simulink model "SMC"  (R2023b)
settings: Solver=VariableStepAuto  StartTime=0.0  StopTime=tf  RelTol=1e-7
values from neighbouring files (symbols this model uses):
  A = Ixx-Kpdot    (= 4100300)    [ShipFinStabilizers.m]
  b = B/A    (= -0.123183501573)    [ShipFinStabilizers.m]    (also in analisi_LUCIA.m = 1)
  B = Kp + Kup - 2*Kalpha*rf/U    (= -505089.3115)    [ShipFinStabilizers.m]
  c = C/A    (= -0.101455991025)    [ShipFinStabilizers.m]
  C = Knl    (= -416000)    [ShipFinStabilizers.m]
  controller_on = 1    [ShipFinStabilizers.m]    (also in off.m = 0; on.m; plotRoutine.m)
  d = D/A    (= -0.0647513596566)    [ShipFinStabilizers.m]    (also in analisi_LUCIA.m = -0.1)
  D = KphiUU*U^2    (= -265500)    [ShipFinStabilizers.m]
  f = F/A    (= -0.00439842816379)    [ShipFinStabilizers.m]
  F = -2*Kalpha    (= -18034.875)    [ShipFinStabilizers.m]
  Fw = 0.2    [ShipFinStabilizers.m]    (also in plotRoutine.m = Fw_vect(i))
  k = 8    [ShipFinStabilizers.m]    (also in analisi_LUCIA.m = 0.25)
  omega_w = 1.3    [ShipFinStabilizers.m]    (also in plotRoutine.m = omega_w_vect(j))
  p1 = 1    [ShipFinStabilizers.m]
  p2 = 2    [ShipFinStabilizers.m]
  rate = 90    [ShipFinStabilizers.m]
  regularizer = 0.1    [ShipFinStabilizers.m]
  sat = 45    [ShipFinStabilizers.m]
  x0 = [deg2rad(20);0]    [ShipFinStabilizers.m]
libraries: simulink x1
settings Model: Creator=valen  LastModifiedBy=valen

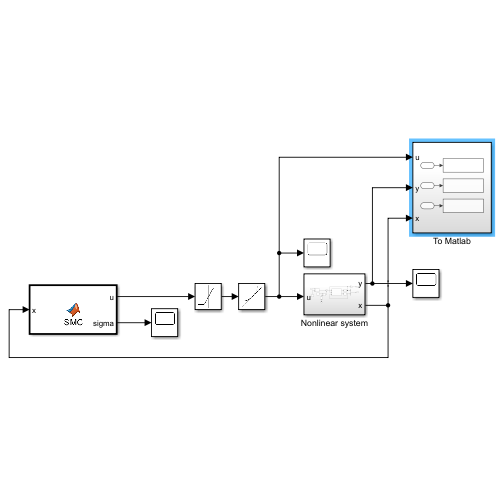
[thumbnail: Simulink's stored preview of the top-level diagram]
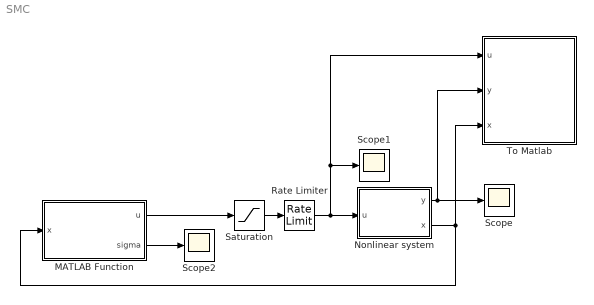
== system SMC ==
  MATLAB Function : MATLAB Function  TreatAsAtomicUnit=on
  Nonlinear system : Subsystem
  Rate Limiter : RateLimiter  RisingSlewLimit=rate  FallingSlewLimit=-rate  SampleTimeMode=inherited
  Saturation : Saturate  UpperLimit=sat  LowerLimit=-sat
  Scope : Scope
  Scope1 : Scope
  Scope2 : Scope
  To Matlab : Subsystem
  wires:
  Rate Limiter/1 -> Scope1/1, To Matlab/1(u), Nonlinear system/1(u)
  Saturation/1 -> Rate Limiter/1
  Nonlinear system/2(x) -> To Matlab/3(x), MATLAB Function/1(x)
  Nonlinear system/1(y) -> To Matlab/2(y), Scope/1
  MATLAB Function/1(u) -> Saturation/1
  MATLAB Function/2(sigma) -> Scope2/1

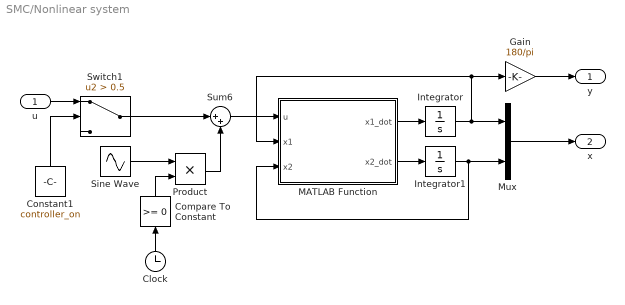
== system SMC/Nonlinear system ==
  u : Inport
  Clock : Clock
  Compare To Constant : simulink/Logic and Bit Operations/Compare To Constant  relop=>=  const=0  OutDataTypeStr=boolean
  Constant1 : Constant  Value=controller_on
  Gain : Gain  Gain=180/pi
  Integrator : Integrator  InitialCondition=x0(1)
  Integrator1 : Integrator  InitialCondition=x0(2)
  MATLAB Function : MATLAB Function  TreatAsAtomicUnit=on
  Mux : Mux  Inputs=2
  Product : Product
  Sine Wave : Sin  Amplitude=Fw/F*A  Frequency=omega_w  SampleTime=0
  Sum6 : Sum  Inputs=|++
  Switch1 : Switch  Criteria=u2 > Threshold  Threshold=0.5  SaturateOnIntegerOverflow=off  InputSameDT=off
  y : Outport
  x : Outport  Port=2
  wires:
  Integrator1/1 -> Mux/2, MATLAB Function/3(x2)
  Integrator/1 -> Mux/1, Gain/1, MATLAB Function/2(x1)
  MATLAB Function/2(x2_dot) -> Integrator1/1
  MATLAB Function/1(x1_dot) -> Integrator/1
  Mux/1 -> x/1
  Sum6/1 -> MATLAB Function/1(u)
  Gain/1 -> y/1
  Constant1/1 -> Switch1/2
  u/1 -> Switch1/1
  Sine Wave/1 -> Product/1
  Switch1/1 -> Sum6/1
  Product/1 -> Sum6/2
  Compare To Constant/1 -> Product/2
  Clock/1 -> Compare To Constant/1

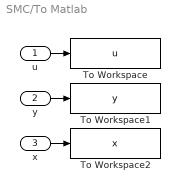
== system SMC/To Matlab ==
  u : Inport  PortDimensions=1
  y : Inport  Port=2  PortDimensions=1
  x : Inport  Port=3  PortDimensions=[2,1]
  To Workspace : ToWorkspace  VariableName=u  SaveFormat=Structure With Time  SampleTime=-1
  To Workspace1 : ToWorkspace  VariableName=y  SaveFormat=Structure With Time  SampleTime=-1
  To Workspace2 : ToWorkspace  VariableName=x  SaveFormat=Structure With Time  SampleTime=-1
  wires:
  y/1 -> To Workspace1/1
  x/1 -> To Workspace2/1
  u/1 -> To Workspace/1

== matlab function SMC/MATLAB Function ==
  data: x input; u output; b parameter; c parameter; d parameter; e parameter; f parameter; p1 parameter; p2 parameter; k parameter; sigma output; regularizer parameter
function [u, sigma] = SMC(x,b, c, d, e, f, p1, p2,k, regularizer)
    
    sigma = p1*x(1) + p2*x(2);
    
    u = -k/p2/f*switching(sigma, regularizer) - ( b*x(2) +c*x(2)*abs(x(2)) + d*x(1) + e*sin(x(1)))/p2/f;
    
end

function s = switching(sigma, regularizer)

    if regularizer>0
        
        %s = tanh(sigma);     

        if sigma <-regularizer
            s = -1;
        elseif sigma > regularizer
            s = +1;
        else
            s = sigma;
        end
        
    else
    
        s = sign(sigma);

    end

end

== matlab function SMC/Nonlinear system/MATLAB Function ==
  data: u input; x1_dot output; x1 input; x2 input; x2_dot output; A parameter; B parameter; C parameter; D parameter; E parameter; F parameter
function [x1_dot,x2_dot] = ship(u,x1,x2, A, B, C, D, E, F)

    x1_dot = x2;
    x2_dot = 1/A*( B*x2 + C*x2*abs(x2) + D*x1 + E*sin(x1) + F*u);
